simulink model "Rr_Variable"  (R2018b)
settings: Solver=VariableStepAuto  StartTime=0.0  StopTime=10.0  RelTol=1e-3
values from neighbouring files (symbols this model uses):
  A = sqrt(2/3)*[1 -0.5 -0.5; 0 sqrt(3)/2 -sqrt(3)/2; sqrt(0.5) sqrt(0.5) sqrt(0.5)]    [MAS_EVV_init.m]
  a1 = input('Reponse : ')    [MAS_EVV_init.m]
  Ai = inv(A)    [MAS_EVV_init.m]
  alfa = 3.98e-3    (= 0.00398)    [MAS_EVV_init.m]
  b1 = input('Reponse : ')    [MAS_EVV_init.m]
  Bi = [1/(sigma*Ls) 0 -Msr/(sigma*Ls*Lr) 0; 0 1/(sigma*Ls) 0 -Msr/(sigma*Ls*Lr); -Msr/(sigma*Ls*Lr) 0 1/(sigma*Ls) 0; 0 -Msr/(sigma*Ls*Lr) 0 1/(sigma*Ls) ]    [MAS_EVV_init.m]
  c1 = input('Reponse : ')    [MAS_EVV_init.m]
  Cn = Pn/Wn    (= 290.939977216)    [MAS_EVV_init.m]    (also in fct_trans.m)
  consi = input('Consigne = ')    [MAS_EVV_init.m]
  consigne = 0    [MAS_EVV_init.m]
  d1 = input('Reponse : ')    [MAS_EVV_init.m]
  delta_T = 80    [MAS_EVV_init.m]
  f = (alpha/100)*Pn/(Wn)^2    (= 0.000141076783904)    [MAS_EVV_init.m]    (also in fct_trans.m)
  J = 0.51    [MAS_EVV_init.m]    (also in fct_trans.m)
  k_couple = 1/(0.3*sigma*Ts)    [MAS_EVV_init.m]    (also in fct_trans.m)
  k_omega = 1/(0.3*0.5)    (= 6.66666666667)    [MAS_EVV_init.m]    (also in fct_trans.m)
  k_phi = 1/(0.3*Tr)    [MAS_EVV_init.m]    (also in fct_trans.m)
  Lr = (N2w/2+L1w)/wn    [MAS_EVV_init.m]    (also in fct_trans.m)
  Ls = (N2w/2+L1w)/wn    [MAS_EVV_init.m]    (also in fct_trans.m)
  Msr = L1w/wn    [MAS_EVV_init.m]    (also in fct_trans.m)
  P = 1    [MAS_EVV_init.m]    (also in fct_trans.m)
  phi_r_n = phi_s_n    (= 1.27323954474)    [MAS_EVV_init.m]    (also in fct_trans.m)
  R0 = Rr/(1+alfa*delta_T)    [MAS_EVV_init.m]
  Rr = double(R2)    [MAS_EVV_init.m]    (also in fct_trans.m)
  Rs = 0.9*Rr    [MAS_EVV_init.m]    (also in fct_trans.m)
  sigma = 1-(Msr^2)/(Ls*Lr)    [MAS_EVV_init.m]    (also in fct_trans.m)
  to = 1    [MAS_EVV_init.m]
  Tr = Lr/Rr    [MAS_EVV_init.m]    (also in fct_trans.m)
  variable = 1    [MAS_EVV_init.m]
  Wb = wn/P    (= 314.159265359)    [MAS_EVV_init.m]    (also in fct_trans.m)
  Wn = 2*pi*Nn/60    (= 309.342156623)    [MAS_EVV_init.m]    (also in fct_trans.m)
  zero_couple = zero(C_couple)    [MAS_EVV_init.m]    (also in fct_trans.m)
  zero_omega = zero(C_omega)    [MAS_EVV_init.m]    (also in fct_trans.m)
  zero_phi = zero(C_phi)    [MAS_EVV_init.m]    (also in fct_trans.m)
undefined symbols (not defined in the file or in its folder): jsin, kcouple, komega, kphi
libraries: powerlib_meascontrol x1
settings Model: Creator=cindyiskandar  LastModifiedBy=cindyiskandar

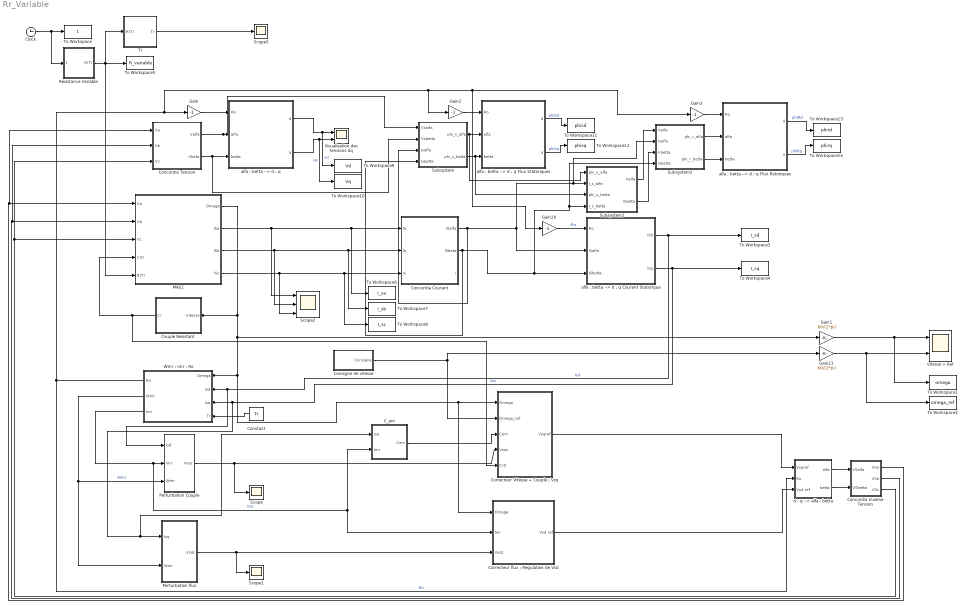
== system Rr_Variable ==
  C_em : Subsystem
  Clock : Clock
  "Concordia Tension " : Subsystem
  "Concordia Courant " : Subsystem
  Concordia Inverse Tension : Subsystem
  Consigne de vitesse : Subsystem
  Constant : Constant  Value=Tr
  Correcteur Vitesse + Couple ; Vsq : Subsystem
  Correcteur flux ; Regulation de Vsd : Subsystem
  Couple Resistant : Subsystem
  Gain{,2..3,20} (4 alike) : Gain  Gain=-1
  Gain1 : Gain  Gain=60/(2*pi)
  Gain21 : Gain  Gain=60/(2*pi)
  MAS1 : Subsystem
  Perturbation Couple : Subsystem
  Perturbation flux : Subsystem
  Resistance Variable : Subsystem
  Scope : Scope
  Scope1 : Scope
  Scope2 : Scope  NumInputPorts=3
  Scope5 : Scope
  Subsystem : Subsystem
  Subsystem1 : Subsystem
  Subsystem2 : Subsystem
  To Workspace : ToWorkspace  VariableName=t  SampleTime=-1
      settings: Save2DSignal=2-D array (concatenate along first dimension)
  To Workspace1 : ToWorkspace  VariableName=omega  SampleTime=-1
      settings: Save2DSignal=2-D array (concatenate along first dimension)
  To Workspace10 : ToWorkspace  VariableName=Vq  SampleTime=-1
      settings: Save2DSignal=2-D array (concatenate along first dimension)
  To Workspace11 : ToWorkspace  VariableName=phisd  SampleTime=-1
      settings: Save2DSignal=2-D array (concatenate along first dimension)
  To Workspace12 : ToWorkspace  VariableName=phisq  SampleTime=-1
      settings: Save2DSignal=2-D array (concatenate along first dimension)
  To Workspace13 : ToWorkspace  VariableName=phird  SampleTime=-1
      settings: Save2DSignal=2-D array (concatenate along first dimension)
  To Workspace14 : ToWorkspace  VariableName=phirq  SampleTime=-1
      settings: Save2DSignal=2-D array (concatenate along first dimension)
  To Workspace2 : ToWorkspace  VariableName=omega_ref  SampleTime=-1
      settings: Save2DSignal=2-D array (concatenate along first dimension)
  To Workspace3 : ToWorkspace  VariableName=I_sd  SampleTime=-1
      settings: Save2DSignal=2-D array (concatenate along first dimension)
  To Workspace4 : ToWorkspace  VariableName=I_sq  SampleTime=-1
      settings: Save2DSignal=2-D array (concatenate along first dimension)
  To Workspace5 : ToWorkspace  VariableName=R_variable  SampleTime=-1
      settings: Save2DSignal=2-D array (concatenate along first dimension)
  To Workspace6 : ToWorkspace  VariableName=I_sa  SampleTime=-1
      settings: Save2DSignal=2-D array (concatenate along first dimension)
  To Workspace7 : ToWorkspace  VariableName=I_sb  SampleTime=-1
      settings: Save2DSignal=2-D array (concatenate along first dimension)
  To Workspace8 : ToWorkspace  VariableName=I_sc  SampleTime=-1
      settings: Save2DSignal=2-D array (concatenate along first dimension)
  To Workspace9 : ToWorkspace  VariableName=Vd  SampleTime=-1
      settings: Save2DSignal=2-D array (concatenate along first dimension)
  Tr : Subsystem
  Visualisation des tensions dq : Scope  NumInputPorts=2
  Vitesse + Ref : Scope  NumInputPorts=2
  Wmr ; Imr ; Ro : Subsystem
  alfa ; betta --> d ; q : Subsystem
  alfa ; betta --> d ; q Courant Statorique : Subsystem
  alfa ; betta --> d ; q Flux Rotoriques : Subsystem
  alfa ; betta --> d ; q Flux Statoriques : Subsystem
  d ; q --> alfa ; betta : Subsystem
  wires:
  "Concordia Courant "/1(ISalfa) -> Subsystem/3(Isalfa), Subsystem2/2(Isalfa), Subsystem1/2(I_s_alfa), alfa ; betta --> d ; q Courant Statorique/2(ISalfa)
  d ; q --> alfa ; betta/2(betta) -> Concordia Inverse Tension/2(VSbetta)
  Subsystem1/2(Irbetta) -> Subsystem2/3(Irbetta)
  Concordia Inverse Tension/2(VSb) -> MAS1/2(Vb), "Concordia Tension "/2("Vb ")
  MAS1/1(Omega) -> Wmr ; Imr ; Ro/1(Omega), Correcteur flux ; Regulation de Vsd/1(Omega), Correcteur Vitesse + Couple ; Vsq/1(Omega), Gain1/1, Couple Resistant/1(Vitesse)
  "Concordia Tension "/1(Valfa) -> Subsystem/1(Vsalfa), alfa ; betta --> d ; q/2(alfa)
  Consigne de vitesse/1(Consigne) -> Correcteur Vitesse + Couple ; Vsq/2(Omega_ref), Gain21/1
  Gain3/1 -> alfa ; betta --> d ; q Flux Rotoriques/1(Ro)
  Subsystem/2(phi_s_betta) -> Subsystem1/3(phi_s_betta), alfa ; betta --> d ; q Flux Statoriques/3("betta ")
  alfa ; betta --> d ; q/1(d) -> To Workspace9/1, Visualisation des tensions dq/1  "vd"
  alfa ; betta --> d ; q/2(q) -> To Workspace10/1, Visualisation des tensions dq/2  "vq"
  Wmr ; Imr ; Ro/1(Ro) -> Gain3/1, Gain20/1, Gain2/1, Gain/1, d ; q --> alfa ; betta/2(Ro)  "Ro"
  Subsystem2/1(phi_r_alfa) -> alfa ; betta --> d ; q Flux Rotoriques/2(alfa)
  Gain1/1 -> To Workspace1/1, Vitesse + Ref/1
  alfa ; betta --> d ; q Courant Statorique/1(ISd) -> Wmr ; Imr ; Ro/2(Isd), Perturbation Couple/1(Isd), To Workspace3/1  "Isd"
  Gain2/1 -> alfa ; betta --> d ; q Flux Statoriques/1(Ro)
  Concordia Inverse Tension/3(VSc) -> MAS1/3(Vc), "Concordia Tension "/3(Vc)
  Gain20/1 -> alfa ; betta --> d ; q Courant Statorique/1(Ro)  "-Ro"
  alfa ; betta --> d ; q Flux Statoriques/2(q) -> To Workspace12/1  "phiSq"
  Correcteur flux ; Regulation de Vsd/1(Vsd ref) -> d ; q --> alfa ; betta/3(Vsd ref)
  MAS1/2(ISa) -> Scope2/1, To Workspace6/1, "Concordia Courant "/1(Ia)
  MAS1/4(ISc) -> Scope2/3, To Workspace8/1, "Concordia Courant "/3(Ic)
  Subsystem/1(phi_s_alfa) -> alfa ; betta --> d ; q Flux Statoriques/2(alfa), Subsystem1/1(phi_s_alfa)
  "Concordia Tension "/2("Vbeta ") -> Subsystem/2(Vsbetta), alfa ; betta --> d ; q/3("betta ")
  Resistance Variable/1(R(T)) -> Tr/1(R(T)), MAS1/5(R(T)), To Workspace5/1
  Perturbation Couple/1("Vsqc ") -> Scope/1, Correcteur Vitesse + Couple ; Vsq/4(Vsqc)
  alfa ; betta --> d ; q Flux Rotoriques/1(d) -> To Workspace13/1  "phiRd"
  d ; q --> alfa ; betta/1(alfa) -> Concordia Inverse Tension/1(VSalfa)
  Wmr ; Imr ; Ro/3(Imr) -> Correcteur flux ; Regulation de Vsd/2(Imr), C_em/2(Imr), Perturbation Couple/2(Imr)  "Imr"
  Clock/1 -> Resistance Variable/1("t "), To Workspace/1
  Concordia Inverse Tension/1(VSa) -> MAS1/1(Va), "Concordia Tension "/1("Va ")
  MAS1/3(ISb) -> Scope2/2, To Workspace7/1, "Concordia Courant "/2(Ib)
  C_em/1(Cem) -> Correcteur Vitesse + Couple ; Vsq/3(Cem)
  Gain/1 -> alfa ; betta --> d ; q/1(Ro)
  Perturbation flux/1(Vsdc) -> Scope1/1, Correcteur flux ; Regulation de Vsd/3(Vsdc)
  alfa ; betta --> d ; q Courant Statorique/2(ISq) -> C_em/1(Isq), Perturbation flux/1(Isq), Wmr ; Imr ; Ro/3(Isq), To Workspace4/1  "Isq"
  Correcteur Vitesse + Couple ; Vsq/1(Vsqref) -> d ; q --> alfa ; betta/1(Vsqref)
  "Concordia Courant "/2("ISbeta ") -> Subsystem/4(Isbetta), Subsystem2/4(Isbetta), Subsystem1/4(I_s_betta), alfa ; betta --> d ; q Courant Statorique/3("ISbetta ")
  Couple Resistant/1(Cr) -> Correcteur Vitesse + Couple ; Vsq/5(Cr0), MAS1/4(Cr0)
  Wmr ; Imr ; Ro/2(Wmr) -> Perturbation flux/2(Wmr), Perturbation Couple/3(Wmr)  "Wmr"
  Tr/1(Tr) -> Scope5/1
  Subsystem2/2(phi_r_betta) -> alfa ; betta --> d ; q Flux Rotoriques/3("betta ")
  Gain21/1 -> To Workspace2/1, Vitesse + Ref/2
  Subsystem1/1(Iralfa) -> Subsystem2/1(Iralfa)
  alfa ; betta --> d ; q Flux Statoriques/1(d) -> To Workspace11/1  "phiSd"
  alfa ; betta --> d ; q Flux Rotoriques/2(q) -> To Workspace14/1  "phiRq"
  Constant/1 -> Wmr ; Imr ; Ro/4(Tr)

== system Rr_Variable/C_em ==
  Isq : Inport
  Imr : Inport  Port=2
  Gain18 : Gain  Gain=P*Msr^2/Lr
  Product13 : Product
  Cem : Outport
  wires:
  Imr/1 -> Product13/1
  Gain18/1 -> Cem/1  "Cem"
  Isq/1 -> Product13/2
  Product13/1 -> Gain18/1

== system Rr_Variable/Concordia Tension  ==
  "Va " : Inport
  "Vb " : Inport  Port=2
  Vc : Inport  Port=3
  Demux : Demux  Outputs=3
  Gain : Gain  Gain=A  Multiplication=Matrix(K*u) (u vector)
  Mux : Mux  Inputs=3
  Valfa : Outport
  "Vbeta " : Outport  Port=2
  wires:
  Demux/1 -> Valfa/1
  "Va "/1 -> Mux/1
  Mux/1 -> Gain/1
  Gain/1 -> Demux/1
  "Vb "/1 -> Mux/2
  Vc/1 -> Mux/3
  Demux/2 -> "Vbeta "/1

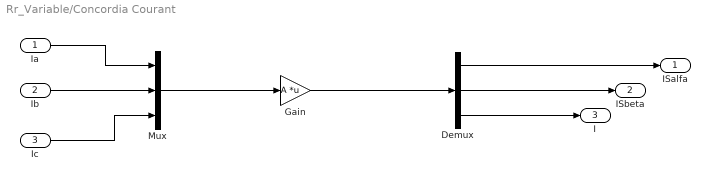
== system Rr_Variable/Concordia Courant  ==
  Ia : Inport
  Ib : Inport  Port=2
  Ic : Inport  Port=3
  Demux : Demux  Outputs=3
  Gain : Gain  Gain=A  Multiplication=Matrix(K*u) (u vector)
  Mux : Mux  Inputs=3
  ISalfa : Outport
  "ISbeta " : Outport  Port=2
  I : Outport  Port=3
  wires:
  Demux/1 -> ISalfa/1
  Ia/1 -> Mux/1
  Mux/1 -> Gain/1
  Gain/1 -> Demux/1
  Ib/1 -> Mux/2
  Ic/1 -> Mux/3
  Demux/2 -> "ISbeta "/1
  Demux/3 -> I/1

== system Rr_Variable/Concordia Inverse Tension ==
  VSalfa : Inport
  VSbetta : Inport  Port=2
  Constant : Constant  Value=0
  Demux : Demux  Outputs=3
  Gain9 : Gain  Gain=Ai  Multiplication=Matrix(K*u) (u vector)
  Mux : Mux  Inputs=3
  VSa : Outport
  VSb : Outport  Port=2
  VSc : Outport  Port=3
  wires:
  Demux/3 -> VSc/1
  Gain9/1 -> Demux/1
  Demux/1 -> VSa/1
  Demux/2 -> VSb/1
  VSbetta/1 -> Mux/2
  VSalfa/1 -> Mux/1
  Mux/1 -> Gain9/1
  Constant/1 -> Mux/3

== system Rr_Variable/Consigne de vitesse ==
  Add : Sum
  Consigne escaliers : powerlib_meascontrol/Pulse & Signal Generators/Stair Generator  t=Tp  e=Omg  Ts=0
      settings: SourceProductName=Simscape Power Systems
  Consigne de Vitesse : Step  After=consi  SampleTime=0
  Gain4 : Gain  Gain=consigne
  Gain5 : Gain  Gain=1-consigne
  Consigne : Outport
  wires:
  Add/1 -> Consigne/1
  Consigne escaliers/1 -> Gain5/1
  Consigne de Vitesse/1 -> Gain4/1
  Gain5/1 -> Add/2
  Gain4/1 -> Add/1

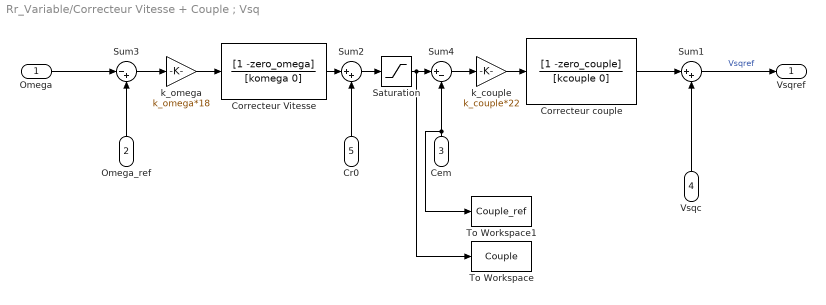
== system Rr_Variable/Correcteur Vitesse + Couple ; Vsq ==
  Omega : Inport
  Omega_ref : Inport  Port=2
  Cem : Inport  Port=3
  Vsqc : Inport  Port=4
  Cr0 : Inport  Port=5
  Correcteur Vitesse : TransferFcn  Numerator=[1 -zero_omega]  Denominator=[komega 0]
  Correcteur couple : TransferFcn  Numerator=[1 -zero_couple]  Denominator=[kcouple 0]
  Saturation : Saturate  UpperLimit=Cn-f*Wn  LowerLimit=-(Cn-f*Wn)
  Sum1 : Sum  Inputs=|++
  Sum2 : Sum  Inputs=|++
  Sum3 : Sum  Inputs=|-+
  Sum4 : Sum  Inputs=|+-
  To Workspace : ToWorkspace  VariableName=Couple  SampleTime=-1
      settings: Save2DSignal=2-D array (concatenate along first dimension)
  To Workspace1 : ToWorkspace  VariableName=Couple_ref  SampleTime=-1
      settings: Save2DSignal=2-D array (concatenate along first dimension)
  k_couple : Gain  Gain=k_couple*22
  k_omega : Gain  Gain=k_omega*18
  Vsqref : Outport
  wires:
  Vsqc/1 -> Sum1/2
  Sum1/1 -> Vsqref/1  "Vsqref"
  Sum3/1 -> k_omega/1
  Omega/1 -> Sum3/1
  k_couple/1 -> Correcteur couple/1
  Omega_ref/1 -> Sum3/2
  Correcteur couple/1 -> Sum1/1
  k_omega/1 -> Correcteur Vitesse/1
  Correcteur Vitesse/1 -> Sum2/1
  Sum2/1 -> Saturation/1
  Cr0/1 -> Sum2/2
  Saturation/1 -> To Workspace/1, Sum4/1
  Sum4/1 -> k_couple/1
  Cem/1 -> To Workspace1/1, Sum4/2

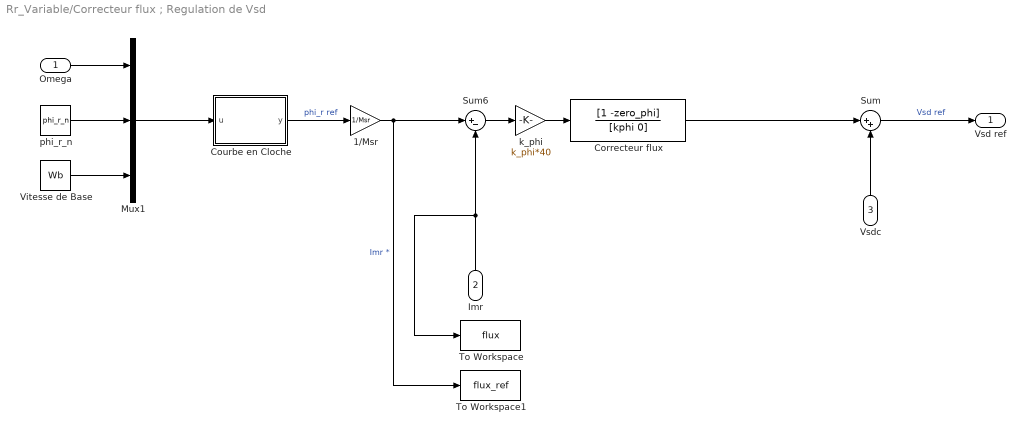
== system Rr_Variable/Correcteur flux ; Regulation de Vsd ==
  Omega : Inport
  Imr : Inport  Port=2
  Vsdc : Inport  Port=3
  1/Msr : Gain  Gain=1/Msr
  Correcteur flux : TransferFcn  Numerator=[1 -zero_phi]  Denominator=[kphi 0]
  Courbe en Cloche : MATLAB Function  TreatAsAtomicUnit=on
  Mux1 : Mux  Inputs=3
  Sum : Sum  Inputs=|++
  Sum6 : Sum  Inputs=|+-
  To Workspace : ToWorkspace  VariableName=flux  SampleTime=-1
      settings: Save2DSignal=2-D array (concatenate along first dimension)
  To Workspace1 : ToWorkspace  VariableName=flux_ref  SampleTime=-1
      settings: Save2DSignal=2-D array (concatenate along first dimension)
  Vitesse de Base : Constant  Value=Wb
  k_phi : Gain  Gain=k_phi*40
  phi_r_n : Constant  Value=phi_r_n
  Vsd ref : Outport
  wires:
  Sum/1 -> Vsd ref/1  "Vsd ref"
  Omega/1 -> Mux1/1
  Courbe en Cloche/1(y) -> 1/Msr/1  "phi_r ref"
  Mux1/1 -> Courbe en Cloche/1(u)
  Sum6/1 -> k_phi/1
  Imr/1 -> To Workspace/1, Sum6/2
  phi_r_n/1 -> Mux1/2
  k_phi/1 -> Correcteur flux/1
  1/Msr/1 -> Sum6/1, To Workspace1/1  "Imr *"
  Vitesse de Base/1 -> Mux1/3
  Correcteur flux/1 -> Sum/1
  Vsdc/1 -> Sum/2

== system Rr_Variable/Couple Resistant ==
  Vitesse : Inport
  Couple Resistant : Subsystem
  "Cr " : Sum  Inputs=++++
  Scope : Scope
  Cr : Outport
  wires:
  "Cr "/1 -> Scope/1, Cr/1  "Cr"
  Couple Resistant/1(Omega^2) -> "Cr "/1
  Vitesse/1 -> Couple Resistant/1(Omega)
  Couple Resistant/4(1/Omega) -> "Cr "/4
  Couple Resistant/3(cte) -> "Cr "/3
  Couple Resistant/2(omega) -> "Cr "/2

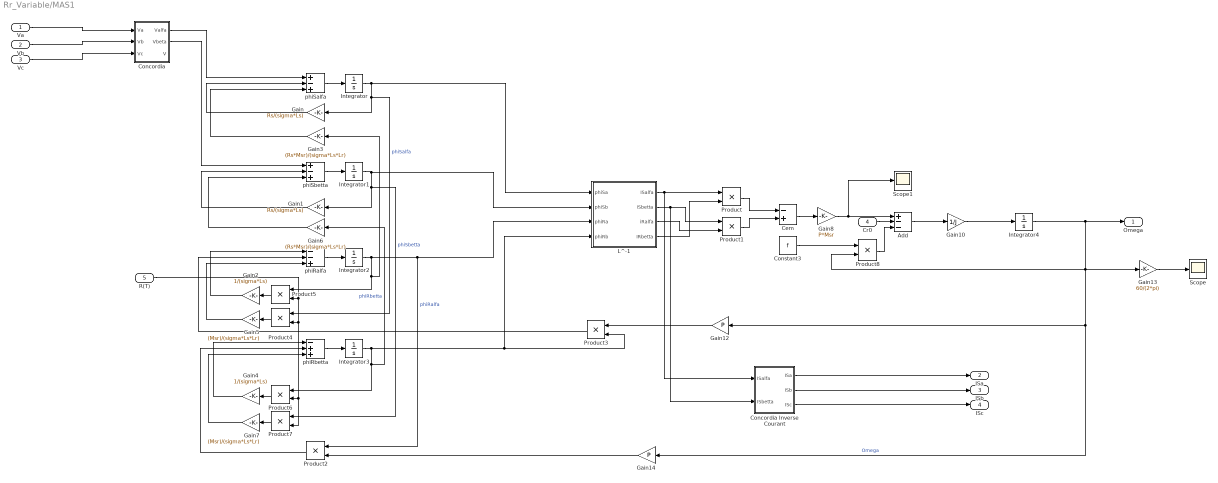
== system Rr_Variable/MAS1 ==
  Va : Inport
  Vb : Inport  Port=2
  Vc : Inport  Port=3
  Cr0 : Inport  Port=4
  R(T) : Inport  Port=5
  Add : Sum  Inputs=+--
  Cem : Sum  Inputs=-+
  "Concordia " : Subsystem
  Concordia Inverse Courant : Subsystem
  Constant3 : Constant  Value=f
  Gain : Gain  Gain=Rs/(sigma*Ls)
  Gain1 : Gain  Gain=Rs/(sigma*Ls)
  Gain10 : Gain  Gain=1/J
  Gain12 : Gain  Gain=P
  Gain13 : Gain  Gain=60/(2*pi)
  Gain14 : Gain  Gain=P
  Gain2 : Gain  Gain=1/(sigma*Ls)
  Gain3 : Gain  Gain=(Rs*Msr)/(sigma*Ls*Lr)
  Gain4 : Gain  Gain=1/(sigma*Ls)
  Gain5 : Gain  Gain=(Msr)/(sigma*Ls*Lr)
  Gain6 : Gain  Gain=(Rs*Msr)/(sigma*Ls*Lr)
  Gain7 : Gain  Gain=(Msr)/(sigma*Ls*Lr)
  Gain8 : Gain  Gain=P*Msr
  Integrator{,1..4} (5 alike) : Integrator
  "L^-1 " : Subsystem
  Product{,1..8} (9 alike) : Product
  Scope : Scope
  Scope1 : Scope
  phiRalfa : Sum  Inputs=--+
  phiRbetta : Sum  Inputs=-++
  phiSalfa : Sum  Inputs=+-+
  phiSbetta : Sum  Inputs=+-+
  Omega : Outport
  ISa : Outport  Port=2
  ISb : Outport  Port=3
  ISc : Outport  Port=4
  wires:
  Vb/1 -> "Concordia "/2("Vb ")
  Va/1 -> "Concordia "/1("Va ")
  phiSbetta/1 -> Integrator1/1
  Concordia Inverse Courant/2(ISb) -> ISb/1
  Concordia Inverse Courant/1(ISa) -> ISa/1
  Gain6/1 -> phiSbetta/3
  Gain8/1 -> Scope1/1, Add/1
  Gain1/1 -> phiSbetta/2
  Gain14/1 -> Product2/2
  Gain10/1 -> Integrator4/1
  Gain12/1 -> Product3/1
  Add/1 -> Gain10/1
  phiSalfa/1 -> Integrator/1
  phiRalfa/1 -> Integrator2/1
  Concordia Inverse Courant/3(ISc) -> ISc/1
  Integrator4/1 -> Gain12/1, Gain14/1, Product8/2, Gain13/1, Omega/1  "Omega"
  phiRbetta/1 -> Integrator3/1
  "L^-1 "/4(IRbetta) -> Product/2
  Cem/1 -> Gain8/1
  "L^-1 "/1(ISalfa) -> Concordia Inverse Courant/1(ISalfa), Product/1
  Gain3/1 -> phiSalfa/3
  "Concordia "/2("Vbeta ") -> phiSbetta/1
  Product3/1 -> phiRalfa/2
  Product/1 -> Cem/1
  Gain/1 -> phiSalfa/2
  "L^-1 "/3(iRalfa) -> Product1/2
  Integrator2/1 -> Product2/1, "L^-1 "/3(phiRa), Product5/1, Gain3/1  "phiRalfa"
  Product1/1 -> Cem/2
  Vc/1 -> "Concordia "/3(Vc)
  Integrator1/1 -> Product7/1, Gain1/1, "L^-1 "/2(phiSb)  "phiSbetta"
  Integrator3/1 -> Product6/1, Gain6/1, "L^-1 "/4(phiRb), Product3/2  "phiRbetta"
  Product2/1 -> phiRbetta/2
  "Concordia "/1(Valfa) -> phiSalfa/1
  "L^-1 "/2(iSbetta) -> Concordia Inverse Courant/2(ISbetta), Product1/1
  Integrator/1 -> Product4/1, Gain/1, "L^-1 "/1(phiSa)  "phiSalfa"
  Gain13/1 -> Scope/1
  Cr0/1 -> Add/2
  Product5/1 -> Gain2/1
  Product4/1 -> Gain5/1
  R(T)/1 -> Product7/2, Product6/2, Product4/2, Product5/2
  Product6/1 -> Gain4/1
  Product7/1 -> Gain7/1
  Constant3/1 -> Product8/1
  Product8/1 -> Add/3
  Gain2/1 -> phiRalfa/1
  Gain5/1 -> phiRalfa/3
  Gain4/1 -> phiRbetta/1
  Gain7/1 -> phiRbetta/3

== system Rr_Variable/Perturbation Couple ==
  Isd : Inport
  Imr : Inport  Port=2
  Wmr : Inport  Port=3
  Add2 : Sum
  Gain15 : Gain  Gain=(1-sigma)*Ls
  Gain17 : Gain  Gain=sigma*Ls
  Product10 : Product
  Product11 : Product
  "Vsqc " : Outport
  wires:
  Add2/1 -> "Vsqc "/1  "Vsqc"
  Product10/1 -> Gain15/1  "Imr*Wmr"
  Imr/1 -> Product10/1
  Gain15/1 -> Add2/1
  Gain17/1 -> Add2/2
  Wmr/1 -> Product11/2, Product10/2
  Isd/1 -> Product11/1
  Product11/1 -> Gain17/1  "Isd*Wmr"

== system Rr_Variable/Perturbation flux ==
  Isq : Inport
  Wmr : Inport  Port=2
  Gain16 : Gain  Gain=-sigma*Ls
  Product9 : Product
  Vsdc : Outport
  wires:
  Isq/1 -> Product9/1
  Wmr/1 -> Product9/2
  Gain16/1 -> Vsdc/1  "Vsdc"
  Product9/1 -> Gain16/1

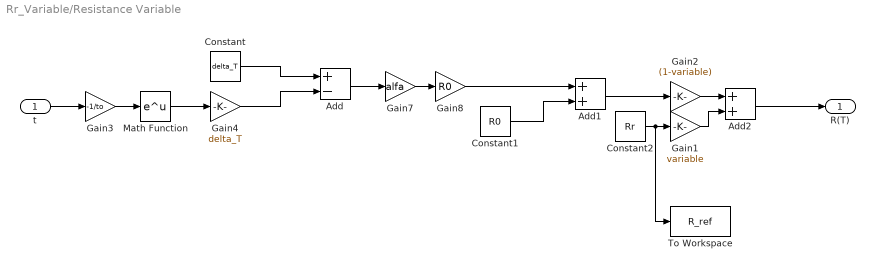
== system Rr_Variable/Resistance Variable ==
  "t " : Inport
  Add : Sum  Inputs=+-
  Add1 : Sum
  Add2 : Sum
  Constant : Constant  Value=delta_T
  Constant1 : Constant  Value=R0
  Constant2 : Constant  Value=Rr
  Gain1 : Gain  Gain=variable
  Gain2 : Gain  Gain=(1-variable)
  Gain3 : Gain  Gain=-1/to
  Gain4 : Gain  Gain=delta_T
  Gain7 : Gain  Gain=alfa
  Gain8 : Gain  Gain=R0
  Math Function : Math  SaturateOnIntegerOverflow=on
  To Workspace : ToWorkspace  VariableName=R_ref  SampleTime=-1
      settings: Save2DSignal=2-D array (concatenate along first dimension)
  R(T) : Outport
  wires:
  "t "/1 -> Gain3/1
  Gain7/1 -> Gain8/1
  Add1/1 -> Gain2/1
  Gain4/1 -> Add/2
  Gain3/1 -> Math Function/1
  Gain8/1 -> Add1/1
  Constant/1 -> Add/1
  Math Function/1 -> Gain4/1
  Constant1/1 -> Add1/2
  Add/1 -> Gain7/1
  Constant2/1 -> To Workspace/1, Gain1/1
  Gain1/1 -> Add2/2
  Gain2/1 -> Add2/1
  Add2/1 -> R(T)/1

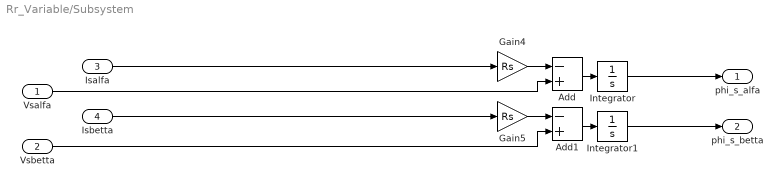
== system Rr_Variable/Subsystem ==
  Vsalfa : Inport
  Vsbetta : Inport  Port=2
  Isalfa : Inport  Port=3
  Isbetta : Inport  Port=4
  Add : Sum  Inputs=-+
  Add1 : Sum  Inputs=-+
  Gain4 : Gain  Gain=Rs
  Gain5 : Gain  Gain=Rs
  Integrator : Integrator
  Integrator1 : Integrator
  phi_s_alfa : Outport
  phi_s_betta : Outport  Port=2
  wires:
  Isbetta/1 -> Gain5/1
  Integrator1/1 -> phi_s_betta/1
  Integrator/1 -> phi_s_alfa/1
  Add1/1 -> Integrator1/1
  Add/1 -> Integrator/1
  Vsalfa/1 -> Add/2
  Gain5/1 -> Add1/1
  Isalfa/1 -> Gain4/1
  Vsbetta/1 -> Add1/2
  Gain4/1 -> Add/1

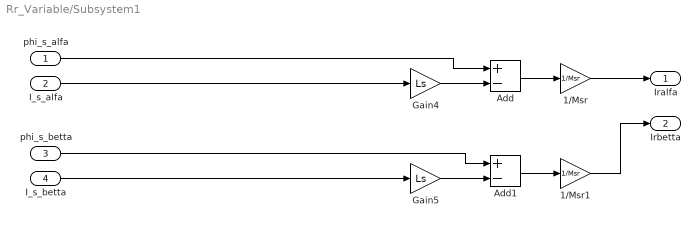
== system Rr_Variable/Subsystem1 ==
  phi_s_alfa : Inport
  I_s_alfa : Inport  Port=2
  phi_s_betta : Inport  Port=3
  I_s_betta : Inport  Port=4
  1/Msr : Gain  Gain=1/Msr
  1/Msr1 : Gain  Gain=1/Msr
  Add : Sum  Inputs=+-
  Add1 : Sum  Inputs=+-
  Gain4 : Gain  Gain=Ls
  Gain5 : Gain  Gain=Ls
  Iralfa : Outport
  Irbetta : Outport  Port=2
  wires:
  phi_s_betta/1 -> Add1/1
  I_s_betta/1 -> Gain5/1
  phi_s_alfa/1 -> Add/1
  I_s_alfa/1 -> Gain4/1
  Add1/1 -> 1/Msr1/1
  1/Msr1/1 -> Irbetta/1
  Gain5/1 -> Add1/2
  1/Msr/1 -> Iralfa/1
  Add/1 -> 1/Msr/1
  Gain4/1 -> Add/2

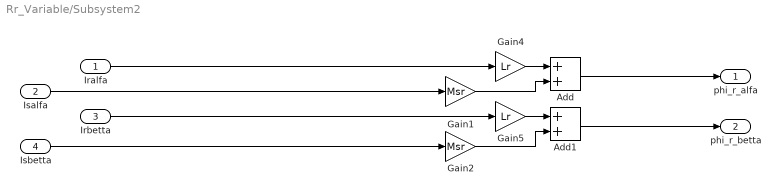
== system Rr_Variable/Subsystem2 ==
  Iralfa : Inport
  Isalfa : Inport  Port=2
  Irbetta : Inport  Port=3
  Isbetta : Inport  Port=4
  Add : Sum
  Add1 : Sum
  Gain1 : Gain  Gain=Msr
  Gain2 : Gain  Gain=Msr
  Gain4 : Gain  Gain=Lr
  Gain5 : Gain  Gain=Lr
  phi_r_alfa : Outport
  phi_r_betta : Outport  Port=2
  wires:
  Irbetta/1 -> Gain5/1
  Add1/1 -> phi_r_betta/1
  Add/1 -> phi_r_alfa/1
  Isalfa/1 -> Gain1/1
  Gain5/1 -> Add1/1
  Iralfa/1 -> Gain4/1
  Isbetta/1 -> Gain2/1
  Gain4/1 -> Add/1
  Gain1/1 -> Add/2
  Gain2/1 -> Add1/2

== system Rr_Variable/Tr ==
  R(T) : Inport
  Constant : Constant  Value=Lr
  Divide : Product  Inputs=*/
  Tr : Outport
  wires:
  Divide/1 -> Tr/1
  Constant/1 -> Divide/1
  R(T)/1 -> Divide/2

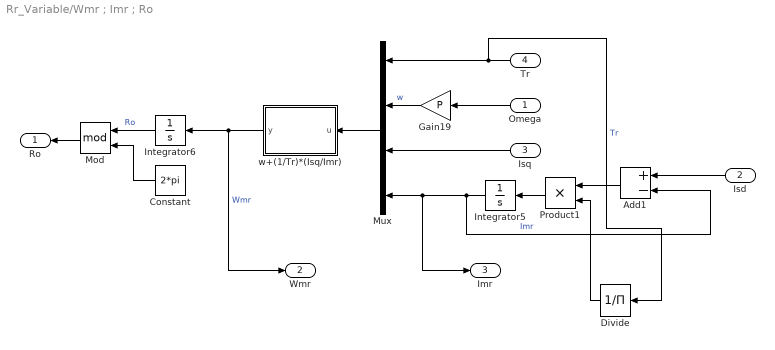
== system Rr_Variable/Wmr ; Imr ; Ro ==
  Omega : Inport
  Isd : Inport  Port=2
  Isq : Inport  Port=3
  Tr : Inport  Port=4
  Add1 : Sum  Inputs=+-
  Constant : Constant  Value=2*pi
  Divide : Product  Inputs=/
  Gain19 : Gain  Gain=P
  Integrator5 : Integrator
  Integrator6 : Integrator
  Mod : Math  Operator=mod  SaturateOnIntegerOverflow=on
  Mux : Mux
  Product1 : Product
  w+(1/Tr)*(Isq/Imr) : MATLAB Function  TreatAsAtomicUnit=on
  Ro : Outport
  Wmr : Outport  Port=2
  Imr : Outport  Port=3
  wires:
  Mod/1 -> Ro/1
  w+(1/Tr)*(Isq/Imr)/1(y) -> Wmr/1, Integrator6/1  "Wmr"
  Integrator6/1 -> Mod/1  "Ro"
  Constant/1 -> Mod/2
  Mux/1 -> w+(1/Tr)*(Isq/Imr)/1(u)
  Gain19/1 -> Mux/2  "w"
  Integrator5/1 -> Add1/2, Imr/1, Mux/4  "Imr"
  Isq/1 -> Mux/3
  Isd/1 -> Add1/1
  Omega/1 -> Gain19/1
  Tr/1 -> Divide/1, Mux/1  "Tr"
  Divide/1 -> Product1/2
  Product1/1 -> Integrator5/1
  Add1/1 -> Product1/1

== system Rr_Variable/alfa ; betta --> d ; q ==
  Ro : Inport
  alfa : Inport  Port=2
  "betta " : Inport  Port=3
  Complex to Real-Imag6 : ComplexToRealImag
  Cos+jSin : Trigonometry  Operator=cos + jsin
  Product14 : Product
  Real-Imag to Complex6 : RealImagToComplex
  d : Outport
  q : Outport  Port=2
  wires:
  alfa/1 -> Real-Imag to Complex6/1
  Product14/1 -> Complex to Real-Imag6/1
  "betta "/1 -> Real-Imag to Complex6/2
  Complex to Real-Imag6/1 -> d/1  "Vd"
  Complex to Real-Imag6/2 -> q/1  "Vq"
  Real-Imag to Complex6/1 -> Product14/2
  Cos+jSin/1 -> Product14/1
  Ro/1 -> Cos+jSin/1

== system Rr_Variable/alfa ; betta --> d ; q Courant Statorique ==
  Ro : Inport
  ISalfa : Inport  Port=2
  "ISbetta " : Inport  Port=3
  Complex to Real-Imag6 : ComplexToRealImag
  Cos+jSin : Trigonometry  Operator=cos + jsin
  Product14 : Product
  Real-Imag to Complex6 : RealImagToComplex
  ISd : Outport
  ISq : Outport  Port=2
  wires:
  ISalfa/1 -> Real-Imag to Complex6/1
  Product14/1 -> Complex to Real-Imag6/1
  "ISbetta "/1 -> Real-Imag to Complex6/2
  Complex to Real-Imag6/1 -> ISd/1  "ISd"
  Complex to Real-Imag6/2 -> ISq/1  "ISq"
  Real-Imag to Complex6/1 -> Product14/2
  Cos+jSin/1 -> Product14/1
  Ro/1 -> Cos+jSin/1

== system Rr_Variable/alfa ; betta --> d ; q Flux Rotoriques ==
  Ro : Inport
  alfa : Inport  Port=2
  "betta " : Inport  Port=3
  Complex to Real-Imag6 : ComplexToRealImag
  Cos+jSin : Trigonometry  Operator=cos + jsin
  Product14 : Product
  Real-Imag to Complex6 : RealImagToComplex
  d : Outport
  q : Outport  Port=2
  wires:
  alfa/1 -> Real-Imag to Complex6/1
  Product14/1 -> Complex to Real-Imag6/1
  "betta "/1 -> Real-Imag to Complex6/2
  Complex to Real-Imag6/1 -> d/1  "phiRd"
  Complex to Real-Imag6/2 -> q/1  "phiRq"
  Real-Imag to Complex6/1 -> Product14/2
  Cos+jSin/1 -> Product14/1
  Ro/1 -> Cos+jSin/1

== system Rr_Variable/alfa ; betta --> d ; q Flux Statoriques ==
  Ro : Inport
  alfa : Inport  Port=2
  "betta " : Inport  Port=3
  Complex to Real-Imag6 : ComplexToRealImag
  Cos+jSin : Trigonometry  Operator=cos + jsin
  Product14 : Product
  Real-Imag to Complex6 : RealImagToComplex
  d : Outport
  q : Outport  Port=2
  wires:
  alfa/1 -> Real-Imag to Complex6/1
  Product14/1 -> Complex to Real-Imag6/1
  "betta "/1 -> Real-Imag to Complex6/2
  Complex to Real-Imag6/1 -> d/1  "phiSd"
  Complex to Real-Imag6/2 -> q/1  "phiSq"
  Real-Imag to Complex6/1 -> Product14/2
  Cos+jSin/1 -> Product14/1
  Ro/1 -> Cos+jSin/1

== system Rr_Variable/d ; q --> alfa ; betta ==
  Vsqref : Inport
  Ro : Inport  Port=2
  Vsd ref : Inport  Port=3
  Complex to Real-Imag5 : ComplexToRealImag
  Cos+jSin1 : Trigonometry  Operator=cos + jsin
  Product12 : Product
  Real-Imag to Complex5 : RealImagToComplex
  alfa : Outport
  betta : Outport  Port=2
  wires:
  Vsqref/1 -> Real-Imag to Complex5/2
  Complex to Real-Imag5/1 -> alfa/1
  Ro/1 -> Cos+jSin1/1
  Vsd ref/1 -> Real-Imag to Complex5/1
  Product12/1 -> Complex to Real-Imag5/1
  Cos+jSin1/1 -> Product12/2  "exp(j*Ro)"
  Real-Imag to Complex5/1 -> Product12/1
  Complex to Real-Imag5/2 -> betta/1

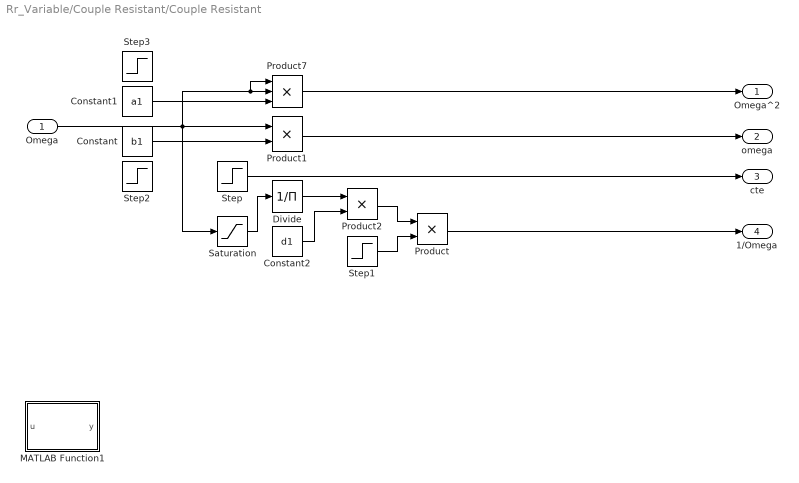
== system Rr_Variable/Couple Resistant/Couple Resistant ==
  Omega : Inport
  Constant : Constant  Value=b1
  Constant1 : Constant  Value=a1
  Constant2 : Constant  Value=d1
  Divide : Product  Inputs=/
  MATLAB Function1 : MATLAB Function  TreatAsAtomicUnit=on
  Product : Product
  Product1 : Product
  Product2 : Product
  Product7 : Product  Inputs=3
  Saturation : Saturate  UpperLimit=Wn  LowerLimit=0.01  OutMin=[0.01]  OutMax=[Wn]
  Step : Step  Time=5  After=c1  SampleTime=0
  Step1 : Step  Time=2  SampleTime=0
  Step2 : Step  Time=2  After=b1  SampleTime=0
  Step3 : Step  Time=2  After=a1  SampleTime=0
  Omega^2 : Outport
  omega : Outport  Port=2
  cte : Outport  Port=3
  1/Omega : Outport  Port=4
  wires:
  Omega/1 -> Saturation/1, Product1/1, Product7/1, Product7/2
  Step/1 -> cte/1
  Product7/1 -> Omega^2/1
  Saturation/1 -> Divide/1
  Product/1 -> 1/Omega/1
  Step1/1 -> Product/2
  Product2/1 -> Product/1
  Divide/1 -> Product2/1
  Constant2/1 -> Product2/2
  Product1/1 -> omega/1
  Constant1/1 -> Product7/3
  Constant/1 -> Product1/2

== system Rr_Variable/MAS1/Concordia  ==
  "Va " : Inport
  "Vb " : Inport  Port=2
  Vc : Inport  Port=3
  Demux : Demux  Outputs=3
  Gain : Gain  Gain=A  Multiplication=Matrix(K*u) (u vector)
  Mux : Mux  Inputs=3
  Valfa : Outport
  "Vbeta " : Outport  Port=2
  V : Outport  Port=3
  wires:
  Demux/1 -> Valfa/1
  "Va "/1 -> Mux/1
  Mux/1 -> Gain/1
  Gain/1 -> Demux/1
  "Vb "/1 -> Mux/2
  Vc/1 -> Mux/3
  Demux/2 -> "Vbeta "/1
  Demux/3 -> V/1

== system Rr_Variable/MAS1/Concordia Inverse Courant ==
  ISalfa : Inport
  ISbetta : Inport  Port=2
  Constant : Constant  Value=0
  Demux : Demux  Outputs=3
  Gain9 : Gain  Gain=Ai  Multiplication=Matrix(K*u) (u vector)
  Mux : Mux  Inputs=3
  ISa : Outport
  ISb : Outport  Port=2
  ISc : Outport  Port=3
  wires:
  Demux/3 -> ISc/1
  Gain9/1 -> Demux/1
  Demux/1 -> ISa/1
  Demux/2 -> ISb/1
  ISbetta/1 -> Mux/2
  ISalfa/1 -> Mux/1
  Mux/1 -> Gain9/1
  Constant/1 -> Mux/3

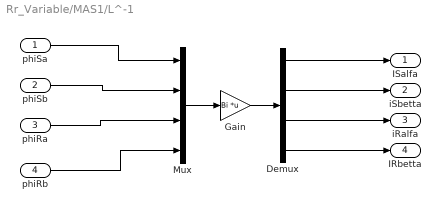
== system Rr_Variable/MAS1/L^-1  ==
  phiSa : Inport
  phiSb : Inport  Port=2
  phiRa : Inport  Port=3
  phiRb : Inport  Port=4
  Demux : Demux
  Gain : Gain  Gain=Bi  Multiplication=Matrix(K*u) (u vector)
  Mux : Mux
  ISalfa : Outport
  iSbetta : Outport  Port=2
  iRalfa : Outport  Port=3
  IRbetta : Outport  Port=4
  wires:
  phiRb/1 -> Mux/4
  Demux/4 -> IRbetta/1
  Mux/1 -> Gain/1
  Gain/1 -> Demux/1
  Demux/1 -> ISalfa/1
  phiSa/1 -> Mux/1
  phiRa/1 -> Mux/3
  Demux/3 -> iRalfa/1
  phiSb/1 -> Mux/2
  Demux/2 -> iSbetta/1

== matlab function Rr_Variable/Correcteur flux ; Regulation de Vsd/Courbe en Cloche ==
  data: u input; y output
function y = fcn(u)
    if (abs(u(1))<=u(3))
        y=u(2);
    else
        y=u(2)*abs(u(3))/abs(u(1));
    end
end

== matlab function Rr_Variable/Wmr ; Imr ; Ro/w+(1//Tr)*(Isq//Imr) ==
  data: u input; y output
function y = fcn(u)
    if (abs(u(4))<1e-6)
        y=0;
    else
        y=u(2)+u(3)/(u(4)*u(1));
    end
end

== matlab function Rr_Variable/Couple Resistant/Couple Resistant/MATLAB Function1 ==
  data: u input; y output
function y = inverse(u)
% if u==0
%     y=1/(0.000001);
% end 
% 
% if u~=0
%     y=1/u;
% end  
y=1/(0.1+u);
